simulink model "lick_filter"  (R2023a)
settings: Solver=VariableStepAuto  StartTime=0.0  StopTime=1800  RelTol=1e-3
settings Model: Creator=craig  LastModifiedBy=craig

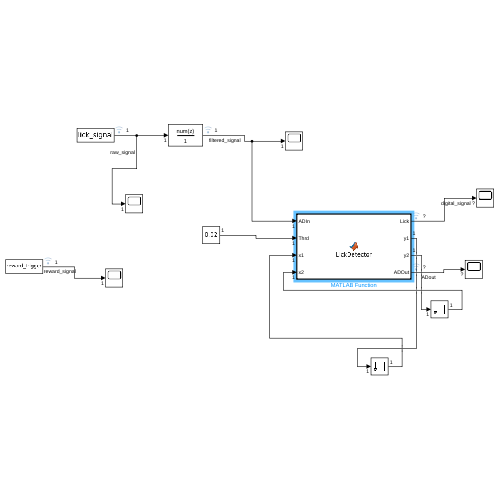
[thumbnail: Simulink's stored preview of the top-level diagram]
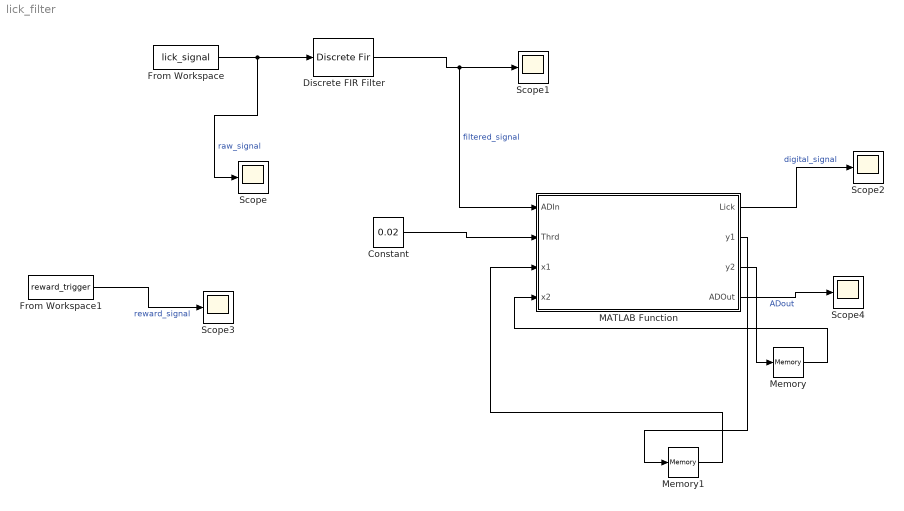
== system lick_filter ==
  Constant : Constant  Value=0.02
  Discrete FIR Filter : DiscreteFir  Coefficients="[0.000509209659813881\t0.000513020363516288\t0.000517670368947169\t0.000523165080954807\t0.000529502229018688\t0.000536671671801312\t0.000544655221147270\t0.000553426486192940\t0.000562950738202937\t0.000573184796705857\t0.000584076937451232\t0.000595566822662082\t0.000607585454003714\t0.000620055148640238\t0.000632889538692870\t0.000645993594362183\t0.000659263670918790\t0.000672587579711404\t0.000685844683282220\t0.000698906014624052\t0.000711634420552287\t0.000723884729108370\t0.000735503940850524\t0.000746331443831085\t0.000756199251997085\t0.000764932266696426\t0.000772348560909980\t0.000778259685775497\t0.000782470998908148\t0.000784782013971788\t0.000784986770893603\t0.000782874226066079\t0.000778228661822321\t0.000770830114425020\t0.000760454819751434\t0.000746875675816741\t0.000729862721224160\t0.000709183628589956\t0.000684604211945086\t0.000655888947078721\t0.000622801503743497\t0.000585105288613380\t0.000542563997844639\t0.000494942178064139\t0.000442005794573363\t0.000383522805539736\t0.000319263740912520\t0.000249002284787882\t0.000172515859925459\t8.95862131054925e-05\t5.45168614075448e-18\t-9.64506317709920e-05\t-0.000199967462741528\t-0.000310745626200165\t-0.000428973038633825\t-0.000554829837350212\t-0.000688487826618691\t-0.000830109933647946\t-0.000979849675716531\t-0.00113785063974888\t-0.00130424597562156\t-0.00147915790444734\t-0.00166269724307814\t-0.00185496294602501\t-0.00205604166597637\t-0.00226600733404635\t-0.00248492076087141\t-0.00271282925961045\t-0.00294976629188174\t-0.00319575113761551\t-0.00345078858976082\t-0.00371486867472770\t-0.00398796639941099\t-0.00427004152556951\t-0.00456103837229735\t-0.00486088564725125\t-0.00516949630725661\t-0.00548676744883370\t-0.00581258022914647\t-0.00614679981779084\t-0.00648927537979570\t-0.00683984009012495\t-0.00719831117991946\t-0.00756449001463563\t-0.00793816220418173\t-0.00831909774507425\t-0.00870705119457714\t-0.00910176187670536\t-0.00950295411992184\t-0.00991033752626848\t-0.0103236072716214\t-0.0107424444366745\t-0.0111665163682081\t-0.0115954770701071\t-0.0120289676235540\t-0.0124666166357312\t-0.0129080407163268\t-0.0133528449810529\t-0.0138006235813448\t-0.0142509602593316\t-0.0147034289271262\t-0.0151575942694157\t-0.0156130123682884\t-0.0160692313491674\t-0.0165257920466955\t-0.0169822286893392\t-0.0174380696014635\t-0.0178928379215595\t-0.0183460523353019\t-0.0187972278220320\t-0.0192458764132781\t-0.0196915079618489\t-0.0201336309200466\t-0.0205717531254864\t-0.0210053825930238\t-0.0214340283112369\t-0.0218572010419305\t-0.0222744141210855\t-0.0226851842596981\t-0.0230890323429240\t-0.0234854842259615\t-0.0238740715250873\t-0.0242543324022972\t-0.0246258123419687\t-0.0249880649180215\t-0.0253406525500261\t-0.0256831472467622\t-0.0260151313357288\t-0.0263361981771474\t-0.0266459528610113\t-0.0269440128857977\t-0.0272300088174485\t-0.0275035849273105\t-0.0277643998077268\t-0.0280121269640498\t-0.0282464553818590\t-0.0284670900682462\t-0.0286737525660541\t-0.0288661814400394\t-0.0290441327339537\t-0.0292073803976255\t-0.0293557166831566\t-0.0294889525094456\t-0.0296069177942718\t-0.0297094617532802\t-0.0297964531652410\t-0.0298677806030557\t-0.0299233526300232\t-0.0299630979609781\t-0.0299869655879580\t2.96949756214538\t-0.0299869655879580\t-0.0299630979609781\t-0.0299233526300232\t-0.0298677806030557\t-0.0297964531652410\t-0.0297094617532802\t-0.0296069177942718\t-0.0294889525094456\t-0.0293557166831566\t-0.0292073803976255\t-0.0290441327339537\t-0.0288661814400394\t-0.0286737525660541\t-0.0284670900682462\t-0.0282464553818590\t-0.0280121269640498\t-0.0277643998077268\t-0.0275035849273105\t-0.0272300088174485\t-0.0269440128857977\t-0.0266459528610113\t-0.0263361981771474\t-0.0260151313357288\t-0.0256831472467622\t-0.0253406525500261\t-0.0249880649180215\t-0.0246258123419687\t-0.0242543324022972\t-0.0238740715250873\t-0.0234854842259615\t-0.0230890323429240\t-0.0226851842596981\t-0.0222744141210855\t-0.0218572010419305\t-0.0214340283112369\t-0.0210053825930238\t-0.0205717531254864\t-0.0201336309200466\t-0.0196915079618489\t-0.0192458764132781\t-0.0187972278220320\t-0.0183460523353019\t-0.0178928379215595\t-0.0174380696014635\t-0.0169822286893392\t-0.0165257920466955\t-0.0160692313491674\t-0.0156130123682884\t-0.0151575942694157\t-0.0147034289271262\t-0.0142509602593316\t-0.0138006235813448\t-0.0133528449810529\t-0.0129080407163268\t-0.0124666166357312\t-0.0120289676235540\t-0.0115954770701071\t-0.0111665163682081\t-0.0107424444366745\t-0.0103236072716214\t-0.00991033752626848\t-0.00950295411992184\t-0.00910176187670536\t-0.00870705119457714\t-0.00831909774507425\t-0.00793816220418173\t-0.00756449001463563\t-0.00719831117991946\t-0.00683984009012495\t-0.00648927537979570\t-0.00614679981779084\t-0.00581258022914647\t-0.00548676744883370\t-0.00516949630725661\t-0.00486088564725125\t-0.00456103837229735\t-0.00427004152556951\t-0.00398796639941099\t-0.00371486867472770\t-0.00345078858976082\t-0.00319575113761551\t-0.00294976629188174\t-0.00271282925961045\t-0.00248492076087141\t-0.00226600733404635\t-0.00205604166597637\t-0.00185496294602501\t-0.00166269724307814\t-0.00147915790444734\t-0.00130424597562156\t-0.00113785063974888\t-0.000979849675716531\t-0.000830109933647946\t-0.000688487826618691\t-0.000554829837350212\t-0.000428973038633825\t-0.000310745626200165\t-0.000199967462741528\t-9.64506317709920e-05\t5.45168614075448e-18\t8.95862131054925e-05\t0.000172515859925459\t0.000249002284787882\t0.000319263740912520\t0.000383522805539736\t0.000442005794573363\t0.000494942178064139\t0.000542563997844639\t0.000585105288613380\t0.000622801503743497\t0.000655888947078721\t0.000684604211945086\t0.000709183628589956\t0.000729862721224160\t0.000746875675816741\t0.000760454819751434\t0.000770830114425020\t0.000778228661822321\t0.000782874226066079\t0.000784986770893603\t0.000784782013971788\t0.000782470998908148\t0.000778259685775497\t0.000772348560909980\t0.000764932266696426\t0.000756199251997085\t0.000746331443831085\t0.000735503940850524\t0.000723884729108370\t0.000711634420552287\t0.000698906014624052\t0.000685844683282220\t0.000672587579711404\t0.000659263670918790\t0.000645993594362183\t0.000632889538692870\t0.000620055148640238\t0.000607585454003714\t0.000595566822662082\t0.000584076937451232\t0.000573184796705857\t0.000562950738202937\t0.000553426486192940\t0.000544655221147270\t0.000536671671801312\t0.000529502229018688\t0.000523165080954807\t0.000517670368947169\t0.000513020363516288\t0.000509209659813881]"
  From Workspace : FromWorkspace  VariableName=lick_signal  SampleTime=0.001
  From Workspace1 : FromWorkspace  VariableName=reward_trigger  SampleTime=0.001
  MATLAB Function : MATLAB Function  TreatAsAtomicUnit=on
  Memory : Memory
  Memory1 : Memory
  Scope{,1..4} (5 alike) : Scope
  wires:
  From Workspace/1 -> Discrete FIR Filter/1, Scope/1  "raw_signal"
  Constant/1 -> MATLAB Function/2(Thrd)
  MATLAB Function/3(y2) -> Memory/1
  Memory/1 -> MATLAB Function/4(x2)
  MATLAB Function/2(y1) -> Memory1/1
  Memory1/1 -> MATLAB Function/3(x1)
  MATLAB Function/1(Lick) -> Scope2/1  "digital_signal"
  From Workspace1/1 -> Scope3/1  "reward_signal"
  Discrete FIR Filter/1 -> MATLAB Function/1(ADIn), Scope1/1  "filtered_signal"
  MATLAB Function/4(ADOut) -> Scope4/1  "ADout"

== matlab function lick_filter/MATLAB Function ==
  data: ADIn input; Lick output; Thrd input; x1 input; x2 input; y1 output; y2 output; ADOut output
function [Lick, y1, y2, ADOut] = LickDetector(ADIn, Thrd, x1, x2)
%#codegen


if ADIn > 0
    ADIn = 0;
end
ADIn = abs(ADIn);

if x1 == 0
    y1 = 0;
end


if ADIn > Thrd
    y1 = x1+1;
    y2 = x2;
else
    y1 = 0;
    y2 = 0;
end

if (y1 >10) && (x2 == 0)
    Lick =1;
    y2 = 1;
else
    Lick = 0;
%    y2 = x2;
end
ADOut = ADIn;
